simulink model "Campus_Power_System"  (R2024a)
settings: Solver=VariableStepAuto  StartTime=0.0  StopTime=0.5  RelTol=1e-3
libraries: spsCurrentMeasurementLib x6, spsVoltageMeasurementLib x6, spsGroundLib x4, spsSeriesRLCLoadLib x3, spsACVoltageSourceLib x3, sps_lib x1, spsThreePhaseTransformerTwoWindingsLib x1
settings Model: Creator=dogba  LastModifiedBy=dogba

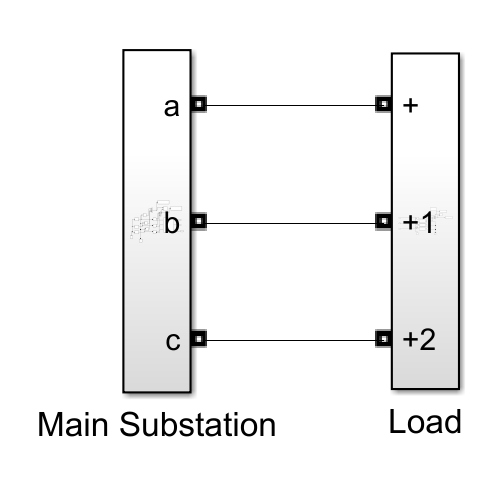
[thumbnail: Simulink's stored preview of the top-level diagram]
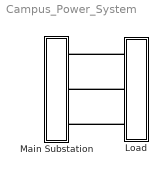
== system Campus_Power_System ==
  Load : Subsystem
  Main Substation : Subsystem
  connections:
  Load/LConn1 -- Main Substation/RConn1
  Load/LConn2 -- Main Substation/RConn2
  Load/LConn3 -- Main Substation/RConn3

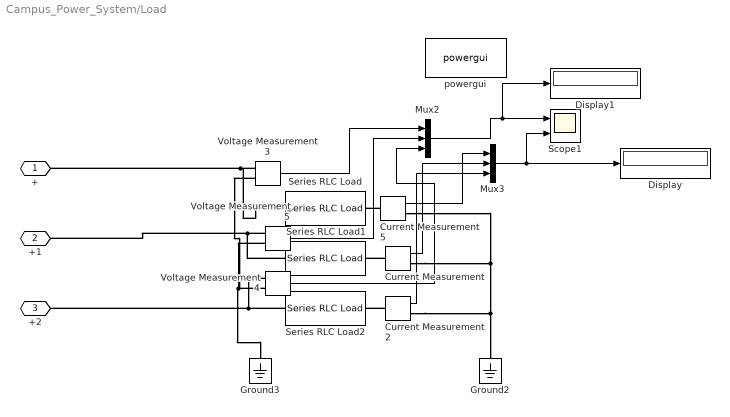
== system Campus_Power_System/Load ==
  Current Measurement : spsCurrentMeasurementLib/Current Measurement  PhasorSimulation=off  OutputType=Complex  PSBequivalent=0
  Current Measurement2 : spsCurrentMeasurementLib/Current Measurement  PhasorSimulation=off  OutputType=Complex  PSBequivalent=0
  Current Measurement5 : spsCurrentMeasurementLib/Current Measurement  PhasorSimulation=off  OutputType=Complex  PSBequivalent=0
  Display : Display
      settings: Format=decimal (Stored Integer)
  Display1 : Display
      settings: Format=decimal (Stored Integer)
  Ground2 : spsGroundLib/Ground  LConnTagsString=a
  Ground3 : spsGroundLib/Ground  LConnTagsString=a
  Mux2 : Mux  Inputs=3
  Mux3 : Mux  Inputs=3
  Scope1 : Scope  NumInputPorts=2
  Series RLC Load : spsSeriesRLCLoadLib/Series RLC Load  LConnTagsString=a  RConnTagsString=__new0  NominalVoltage=300  NominalFrequency=50  ActivePower=10e3  InductivePower=100  CapacitivePower=100  Setx0=off  InitialVoltage=0  SetiL0=off  InitialCurrent=0  Measurements=None  LoadType=constant Z
  Series RLC Load1 : spsSeriesRLCLoadLib/Series RLC Load  LConnTagsString=a  RConnTagsString=__new0  NominalVoltage=250  NominalFrequency=50  ActivePower=10e3  InductivePower=100  CapacitivePower=100  Setx0=off  InitialVoltage=0  SetiL0=off  InitialCurrent=0  Measurements=None  LoadType=constant Z
  Series RLC Load2 : spsSeriesRLCLoadLib/Series RLC Load  LConnTagsString=a  RConnTagsString=__new0  NominalVoltage=220  NominalFrequency=50  ActivePower=10e3  InductivePower=100  CapacitivePower=100  Setx0=off  InitialVoltage=0  SetiL0=off  InitialCurrent=0  Measurements=None  LoadType=constant Z
  Voltage Measurement3 : spsVoltageMeasurementLib/Voltage Measurement  PhasorSimulation=off  OutputType=Complex  PSBequivalent=0
  Voltage Measurement4 : spsVoltageMeasurementLib/Voltage Measurement  PhasorSimulation=off  OutputType=Complex  PSBequivalent=0
  Voltage Measurement5 : spsVoltageMeasurementLib/Voltage Measurement  PhasorSimulation=off  OutputType=Complex  PSBequivalent=0
  powergui : sps_lib/powergui  Priority=1  SimulationMode=Continuous  SampleTime=50e-6  frequency=60  Iterations=50  frequencyindice=50  Pbase=100e6  ErrMax=1e-4  UnitsV=kV  UnitsW=MW  buscounter=0  FunctionMessages=off  echomessages=off  EnableUseOfTLC=off  CurrentSourceSwitches=off  DisableSnubberDevices=off  DisableRonSwitches=off  DisableVfSwitches=off  DisplayEquations=off  AutomaticDiscreteSolvers=off  SolverType=Tustin/Backward Euler (TBE)  Interpol=off  ExternalGateDelay=off  methode=off  Ts=100  x0status=blocks  SPID=on  SwTol=0  HookPort=off  NonlinearTolerance=1e-4  nMaxIteration=100  ContinueOnMaxIteration=off  RestoreLinks=warning  ResistiveCurrentMeasurement=off  Frange=[0:2:500]  Ylog=off  Xlog=on  ShowGrid=off  save=off  variable=ZData  structure=0  ZoomFFT=off  StartTime=0.0  cycles=1  DisplayStyle=1  fundamental=60  FreqAxis=off  MaxFrequency=1000  frequencyindicesteady=1  RmsSteady=1  display=off
  + : PMIOPort  Side=Left
  +1 : PMIOPort  Port=2  Side=Left
  +2 : PMIOPort  Port=3  Side=Left
  wires:
  Current Measurement/1 -> Mux3/2
  Mux2/1 -> Display1/1, Scope1/1
  Voltage Measurement4/1 -> Mux2/3
  Mux3/1 -> Scope1/2, Display/1
  Current Measurement5/1 -> Mux3/1
  Current Measurement2/1 -> Mux3/3
  Voltage Measurement3/1 -> Mux2/1
  Voltage Measurement5/1 -> Mux2/2
  connections:
  Current Measurement5/RConn1 -- Current Measurement/RConn1 -- Current Measurement2/RConn1 -- Ground2/LConn1
  Current Measurement2/LConn1 -- Series RLC Load2/RConn1
  Series RLC Load1/LConn1 -- +1/RConn1 -- Voltage Measurement5/LConn1
  Series RLC Load2/LConn1 -- +2/RConn1 -- Voltage Measurement4/LConn1
  Series RLC Load/LConn1 -- +/RConn1 -- Voltage Measurement3/LConn1
  Current Measurement5/LConn1 -- Series RLC Load/RConn1
  Voltage Measurement4/LConn2 -- Voltage Measurement3/LConn2 -- Voltage Measurement5/LConn2 -- Ground3/LConn1
  Current Measurement/LConn1 -- Series RLC Load1/RConn1

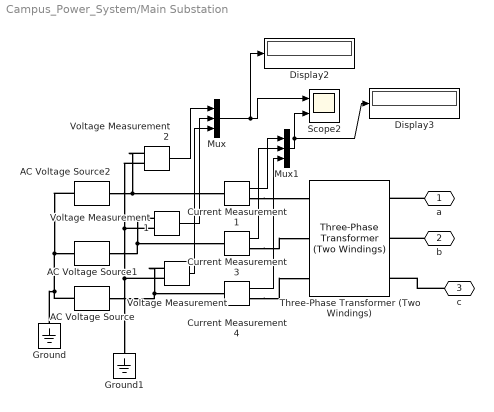
== system Campus_Power_System/Main Substation ==
  AC Voltage Source : spsACVoltageSourceLib/AC Voltage Source  Amplitude=11000  Phase=-120  Frequency=50  SampleTime=0  Measurements=None  BusType=swing  Pref=10e3  Qref=0  Qmin=-inf  Qmax=+inf
  AC Voltage Source1 : spsACVoltageSourceLib/AC Voltage Source  Amplitude=11000  Phase=120  Frequency=50  SampleTime=0  Measurements=None  BusType=swing  Pref=10e3  Qref=0  Qmin=-inf  Qmax=+inf
  AC Voltage Source2 : spsACVoltageSourceLib/AC Voltage Source  Amplitude=11000  Phase=0  Frequency=50  SampleTime=0  Measurements=None  BusType=swing  Pref=10e3  Qref=0  Qmin=-inf  Qmax=+inf
  Current Measurement1 : spsCurrentMeasurementLib/Current Measurement  PhasorSimulation=off  OutputType=Complex  PSBequivalent=0
  Current Measurement3 : spsCurrentMeasurementLib/Current Measurement  PhasorSimulation=off  OutputType=Complex  PSBequivalent=0
  Current Measurement4 : spsCurrentMeasurementLib/Current Measurement  PhasorSimulation=off  OutputType=Complex  PSBequivalent=0
  Display2 : Display
      settings: Format=decimal (Stored Integer)
  Display3 : Display
      settings: Format=decimal (Stored Integer)
  Ground : spsGroundLib/Ground  LConnTagsString=a
  Ground1 : spsGroundLib/Ground  LConnTagsString=a
  Mux : Mux  Inputs=3
  Mux1 : Mux  Inputs=3
  Scope2 : Scope  NumInputPorts=2
  Three-Phase Transformer (Two Windings) : spsThreePhaseTransformerTwoWindingsLib/Three-Phase Transformer (Two Windings)  Winding1Connection=Yg  Winding2Connection=Yg  CoreType=Three single-phase transformers  SetSaturation=off  Hysteresis=off  DataFile='hysteresis'  SetInitialFlux=off  Measurements=None  UNITS=pu  NominalPower=[ 5000e3, 60 ]  Winding1=[11000, 0.002 , 0.08 ]  Winding2=[ 480 , 0.002 , 0.08 ]  Rm=500  Lm=500  L0=0.5  Saturation=[ 0,0 ; 0.0024,1.2 ; 1.0,1.52 ]  InitialFluxes=[ 0.8 , -0.8 , 0.7 ]  BreakLoop=off  DiscreteSolver=Trapezoidal iterative  DataType=off  TransfoNumber=1
  Voltage Measurement : spsVoltageMeasurementLib/Voltage Measurement  PhasorSimulation=off  OutputType=Complex  PSBequivalent=0
  Voltage Measurement1 : spsVoltageMeasurementLib/Voltage Measurement  PhasorSimulation=off  OutputType=Complex  PSBequivalent=0
  Voltage Measurement2 : spsVoltageMeasurementLib/Voltage Measurement  PhasorSimulation=off  OutputType=Complex  PSBequivalent=0
  a : PMIOPort  Side=Right
  b : PMIOPort  Port=2  Side=Right
  c : PMIOPort  Port=3  Side=Right
  wires:
  Current Measurement3/1 -> Mux1/2
  Voltage Measurement1/1 -> Mux/2
  Current Measurement4/1 -> Mux1/3
  Voltage Measurement/1 -> Mux/3
  Voltage Measurement2/1 -> Mux/1
  Current Measurement1/1 -> Mux1/1
  Mux1/1 -> Display3/1, Scope2/2
  Mux/1 -> Display2/1, Scope2/1
  connections:
  AC Voltage Source/LConn1 -- Ground/LConn1 -- AC Voltage Source2/LConn1 -- AC Voltage Source1/LConn1
  AC Voltage Source1/RConn1 -- Voltage Measurement1/LConn1 -- Current Measurement3/LConn1
  Voltage Measurement2/LConn2 -- Voltage Measurement1/LConn2 -- Voltage Measurement/LConn2 -- Ground1/LConn1
  Current Measurement4/RConn1 -- Three-Phase Transformer (Two Windings)/LConn3
  AC Voltage Source/RConn1 -- Voltage Measurement/LConn1 -- Current Measurement4/LConn1
  AC Voltage Source2/RConn1 -- Voltage Measurement2/LConn1 -- Current Measurement1/LConn1
  Current Measurement3/RConn1 -- Three-Phase Transformer (Two Windings)/LConn2
  c/RConn1 -- Three-Phase Transformer (Two Windings)/RConn3
  Current Measurement1/RConn1 -- Three-Phase Transformer (Two Windings)/LConn1
  a/RConn1 -- Three-Phase Transformer (Two Windings)/RConn1
  b/RConn1 -- Three-Phase Transformer (Two Windings)/RConn2
